simulink model "sml_quadrotor"  (R2016a)
settings: Solver=VariableStepAuto  StartTime=0.0  StopTime=10  RelTol=1e-3
undefined symbols (not defined in the file or in its folder): quad
settings Model: Creator=Duy Nam  LastModifiedBy=Duy Nam

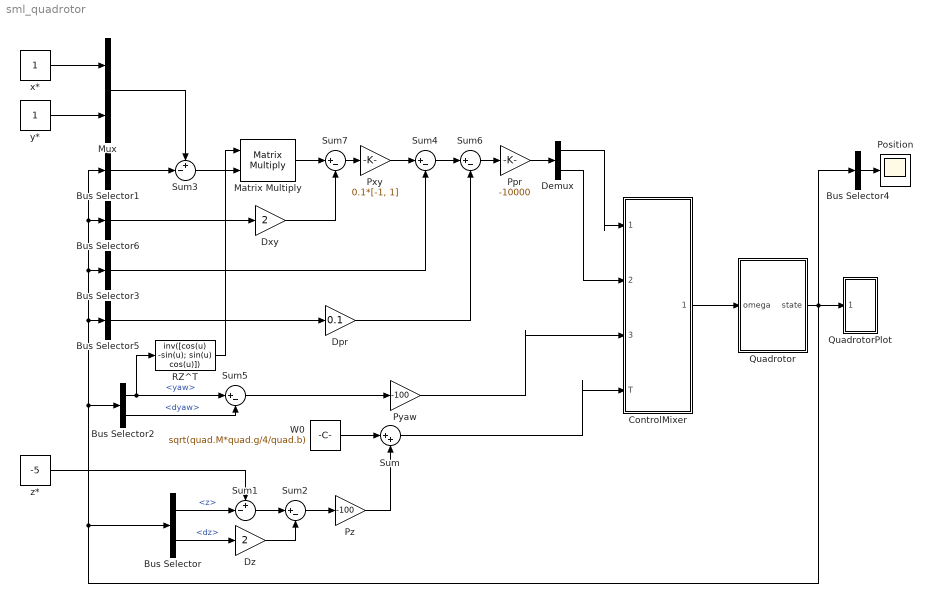
== system sml_quadrotor ==
  Bus Selector : BusSelector  OutputSignals=z,dz
  Bus Selector1 : BusSelector  OutputSignals=x,y  OutputAsBus=on
  Bus Selector2 : BusSelector  OutputSignals=yaw,dyaw
  Bus Selector3 : BusSelector  OutputSignals=pitch,roll  OutputAsBus=on
  Bus Selector4 : BusSelector  OutputSignals=x,y,z  OutputAsBus=on
  Bus Selector5 : BusSelector  OutputSignals=dpitch,droll  OutputAsBus=on
  Bus Selector6 : BusSelector  OutputSignals=dx,dy  OutputAsBus=on
  ControlMixer : Subsystem
  Demux : Demux  Outputs=2
  Dpr : Gain  Gain=0.1
  Dxy : Gain  Gain=2
  Dz : Gain  Gain=2
  Matrix Multiply : Product  Multiplication=Matrix(*)  RndMeth=Zero
  Mux : Mux  Inputs=2
  Position : Scope
  Ppr : Gain  Gain=-10000
  Pxy : Gain  Gain=0.1*[-1, 1]
  Pyaw : Gain  Gain=-100
  Pz : Gain  Gain=-100
  Quadrotor : Subsystem
  QuadrotorPlot : Subsystem
  RZ^T : MATLABFcn  MATLABFcn=inv([cos(u) -sin(u); sin(u) cos(u)])  OutputDimensions=[2 2]  Output1D=off
  Sum : Sum  Inputs=|++
  Sum1 : Sum  Inputs=+-|
  Sum{2,4..7} (5 alike) : Sum  Inputs=|+-
  Sum3 : Sum  Inputs=+-|
  W0 : Constant  Value=sqrt(quad.M*quad.g/4/quad.b)
  x* : Constant
  y* : Constant
  z* : Constant  Value=-5
  wires:
  ControlMixer/1(omega) -> Quadrotor/1(omega)
  RZ^T/1 -> Matrix Multiply/1
  Sum/1 -> ControlMixer/4(T)
  W0/1 -> Sum/1
  z*/1 -> Sum1/1
  Sum2/1 -> Pz/1
  Pz/1 -> Sum/2
  Bus Selector/1 -> Sum1/2  "<z>"
  Sum1/1 -> Sum2/1
  Bus Selector/2 -> Dz/1  "<dz>"
  Dz/1 -> Sum2/2
  x*/1 -> Mux/1
  y*/1 -> Mux/2
  Mux/1 -> Sum3/1
  Bus Selector1/1 -> Sum3/2
  Bus Selector2/1 -> Sum5/1, RZ^T/1  "<yaw>"
  Sum3/1 -> Matrix Multiply/2
  Pxy/1 -> Sum4/1
  Bus Selector3/1 -> Sum4/2
  Sum4/1 -> Sum6/1
  Ppr/1 -> Demux/1
  Demux/2 -> ControlMixer/2(tau_roll)
  Demux/1 -> ControlMixer/1(tau_pitch)
  Bus Selector4/1 -> Position/1
  Pyaw/1 -> ControlMixer/3(tau_yaw)
  Sum5/1 -> Pyaw/1
  Bus Selector2/2 -> Sum5/2  "<dyaw>"
  Sum6/1 -> Ppr/1
  Bus Selector5/1 -> Dpr/1
  Dpr/1 -> Sum6/2
  Quadrotor/1(state) -> Bus Selector4/1, Bus Selector6/1, Bus Selector1/1, Bus Selector3/1, Bus Selector5/1, Bus Selector2/1, Bus Selector/1, QuadrotorPlot/1(state)
  Bus Selector6/1 -> Dxy/1
  Dxy/1 -> Sum7/2
  Matrix Multiply/1 -> Sum7/1
  Sum7/1 -> Pxy/1

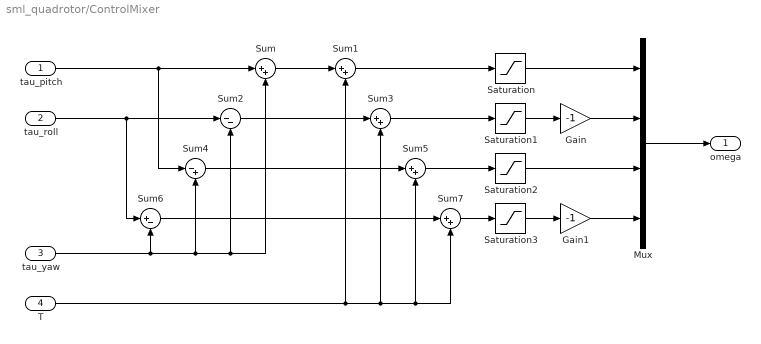
== system sml_quadrotor/ControlMixer ==
  tau_pitch : Inport
  tau_roll : Inport  Port=2
  tau_yaw : Inport  Port=3
  T : Inport  Port=4
  Gain : Gain  Gain=-1
  Gain1 : Gain  Gain=-1
  Mux : Mux
  Saturation{,1..3} (4 alike) : Saturate  UpperLimit=1000  LowerLimit=700
  Sum{,1,3,5,7} (5 alike) : Sum  Inputs=|++
  Sum2 : Sum  Inputs=|--
  Sum4 : Sum  Inputs=|-+
  Sum6 : Sum  Inputs=|+-
  omega : Outport
  wires:
  Sum5/1 -> Saturation2/1
  Saturation2/1 -> Mux/3
  Gain/1 -> Mux/2
  tau_yaw/1 -> Sum/2, Sum2/2, Sum4/2, Sum6/2
  Sum3/1 -> Saturation1/1
  Mux/1 -> omega/1
  Sum/1 -> Sum1/1
  T/1 -> Sum5/2, Sum7/2, Sum3/2, Sum1/2
  Sum7/1 -> Saturation3/1
  Sum2/1 -> Sum3/1
  Sum1/1 -> Saturation/1
  Saturation1/1 -> Gain/1
  Sum4/1 -> Sum5/1
  Gain1/1 -> Mux/4
  tau_pitch/1 -> Sum4/1, Sum/1
  Sum6/1 -> Sum7/1
  tau_roll/1 -> Sum6/1, Sum2/1
  Saturation/1 -> Mux/1
  Saturation3/1 -> Gain1/1

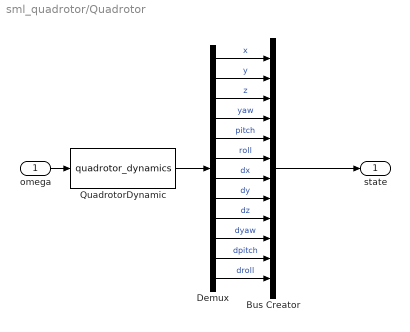
== system sml_quadrotor/Quadrotor ==
  omega : Inport
  Bus Creator : BusCreator  Inputs='x','y','z','yaw','pitch','roll','dx','dy','dz','dyaw','dpitch','droll'
  Demux : Demux  Outputs=12
  QuadrotorDynamic : S-Function  FunctionName=quadrotor_dynamics  Parameters=quad  SFunctionDeploymentMode=off  EnableBusSupport=off
  state : Outport
  wires:
  omega/1 -> QuadrotorDynamic/1
  Demux/8 -> Bus Creator/8  "dy"
  Demux/10 -> Bus Creator/10  "dyaw"
  Demux/3 -> Bus Creator/3  "z"
  Demux/6 -> Bus Creator/6  "roll"
  Demux/5 -> Bus Creator/5  "pitch"
  Demux/1 -> Bus Creator/1  "x"
  Demux/2 -> Bus Creator/2  "y"
  Demux/7 -> Bus Creator/7  "dx"
  Demux/11 -> Bus Creator/11  "dpitch"
  Demux/4 -> Bus Creator/4  "yaw"
  Demux/9 -> Bus Creator/9  "dz"
  Bus Creator/1 -> state/1
  Demux/12 -> Bus Creator/12  "droll"
  QuadrotorDynamic/1 -> Demux/1

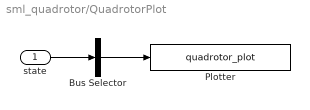
== system sml_quadrotor/QuadrotorPlot ==
  state : Inport
  Bus Selector : BusSelector  OutputSignals=x,y,z,yaw,pitch,roll  OutputAsBus=on
  Plotter : S-Function  FunctionName=quadrotor_plot  Parameters=[2, 10], 1, 1, quad  SFunctionDeploymentMode=off  EnableBusSupport=off
  wires:
  Bus Selector/1 -> Plotter/1
  state/1 -> Bus Selector/1
